simulink model "Commando2"  (R2012b)
settings: Solver=ode5  StartTime=0.0  StopTime=inf  FixedStep=sample_time  RelTol=1e-3
InitFcn:
  | sample_time=0.005;%0.004;%0.0025;%0.02;
  | sample_time_Vicon = 0.005;
  | DeltaT = 0.02;
  | g = 9.81;
  | H0 = g%0.3165;
  | Kl = 1;
  | 
  | Q6_mass = 0.8;
  | 
  | Q6_Omega_r = 1.2; %for horizon ref
  | Q6_Zeta_r = 0.707; %for horizon ref
  | Q6_Omega_r_h = 2;%for vertical ref
  | Q6_Zeta_r_h = 0.7; %for vertical ref
  | 
  | 
  | Q6_Omega = 1.3; %for horizon control
  | Q6_Zeta = 0.707; %for horizon control
  | Q6_Omega_h= 2; %for vertical control
  | Q6_Zeta_h = 0.7; %for vertical control
  | 
  | 
  | Q6_acc_max = 5;%horizontal max acc
  | Q6_acc_max_h = 5;%horizontal max acc
  | 
  | omega_circle = 30*pi/180;
  | 
  | omega_h = 0.1;%Ascending speed
  | PI = pi;
  | Circle_R = 1.9;
  | 
  | 
  | MAX_Height = -2;
  | 
  | 
  | % for NN
  | n = 5;
  | r = 3;
  | n2 = 5;
  | NN_ST = 0.02;
  | 
  | GAMA_V = 6;
  | gama_V_e = 0.01;
  | 
  | GAMA_W = GAMA_V;
  | gama_W_e =0.01;
  | 
  | % deadzone
  | NN_Deadzone_Z = 0;
  | 
  | % inputs nomalizaton parameters
  | NN_Z_y_min = -3;
  | NN_Z_y_max = 0.5;
  | 
  | NN_Z_v_max = 8;
  | NN_Z_v_min = -NN_Z_v_max;
  | 
  | % alpha = 0.034;
  | alpha = 1;
  | % c_f = 0.0015;
  | c_f = 0.001;
  | ... (+1 lines)
libraries: X330_Control x20, simulink x10
(part 2 of 2)

== stateflow chart Commando2/UAV 4/Trajectory Logic/UAV4 SF ==
  state Airborne
    state StopPoint2
      en:PosDesired = Pos;
    state TakeOff
      du:HoverThrottle = (H0 - HoverThrottle)*2*DeltaT + HoverThrottle ;
      PosDesired[2] = (-1.2 - PosDesired[2])*1*DeltaT + PosDesired[2] ;
    state StartPoint1
      en:PosDesired[0] = Circle_R*sin(270*PI/180 );
      PosDesired[1] = Circle_R*cos(270*PI/180);
    state StopPoint
      en:PosDesired = Pos;
      PosDesired[2]=-3;
    state StopPoint1
      en:
      PosDesired[0]=-2.2;
      PosDesired[1]=-2;
    state Circle2D
      du: PosDesired[0] = Circle_R*sin(270*PI/180 + T_circle*omega_circle);
      PosDesired[1] = Circle_R*cos(270*PI/180 + T_circle*omega_circle);
      PosDesired[2]=height;
      T_circle = T_circle + DeltaT;
    (default) -> TakeOff : {PosDesired = Pos; }
    Circle2D -> StopPoint2 [order 1] : [QD==1]
    StopPoint2 -> Circle2D : [QD==0]
    TakeOff -> StartPoint1 : after(10, sec)
    StartPoint1 -> Circle2D : [RC[5] > 0.5]
        | {T_circle = 0.0;}
    Circle2D -> StopPoint [order 2] : [RC[5] < 0.5]
    StopPoint -> StopPoint1 : after (3,sec)
  state Landing
    state Decsending
      en:PosDesired = Pos;
      du:PosDesired[2] = (0.2 - PosDesired[2])*1*DeltaT + PosDesired[2] ;
    state CutThrottle
      du:HoverThrottle = (0.0 - HoverThrottle)*5*DeltaT + HoverThrottle ;
    (default) -> Decsending
    Decsending -> CutThrottle : [Pos[2] > -0.2]
  Landing -> Airborne : [RC[6] > 0.5]
  Airborne -> Landing : [RC[6] < -0.5]
  (default) -> Landing : {HoverThrottle=0.0;}
  data: PosDesired output double size=4; HoverThrottle output double size=1; Mode output uint8 size=3; RC input size=8; Pos input size=4; height input size=1; DeltaT parameter size=1; H0 parameter size=1; Kl parameter size=1; VelCmd local double size=2 =0; line_count local int8 size=1 =0; triangle_count local int8 size=1 =0; T_circle local double size=1; omega_circle parameter size=1; PI parameter size=1; omega_h parameter size=1; Circle_R parameter size=1; MAX_Height parameter size=1; PosError output double; QD input double size=1

== stateflow chart Commando2/UAV 1/Trajectory Logic/UAV SF1 ==
  state Airborne
    state StopPoint2
      en:PosDesired = Pos;
    state TakeOff
      du:HoverThrottle = (H0 - HoverThrottle)*2*DeltaT + HoverThrottle ;
      PosDesired[2] = (-1.2 - PosDesired[2])*1*DeltaT + PosDesired[2] ;
    state StartPoint1
      en:PosDesired[0] = Circle_R*sin(0*PI/180 );
      PosDesired[1] = Circle_R*cos(0*PI/180);
    state StopPoint
      en:PosDesired = Pos;
      PosDesired[2]=-1.5;
    state Circle2D
      du: PosDesired[0] = Circle_R*sin(0*PI/180 + T_circle*omega_circle);
      PosDesired[1] = Circle_R*cos(0*PI/180 + T_circle*omega_circle);
      PosDesired[2]=height;
      T_circle = T_circle + DeltaT;
    state StopPoint1
      en:
      PosDesired[0]=-2.2;
      PosDesired[1]=1;
    (default) -> TakeOff : {PosDesired = Pos; }
    Circle2D -> StopPoint2 [order 1] : [QD==1]
    TakeOff -> StartPoint1 : after(5, sec)
    StopPoint2 -> Circle2D : [QD==0]
    StartPoint1 -> Circle2D : [RC[5] > 0.5]
        | {T_circle = 0.0;}
    Circle2D -> StopPoint [order 2] : [RC[5] < 0.5]
    StopPoint -> StopPoint1 : after (3, sec)
  state Landing
    state Decsending
      en:PosDesired = Pos;
      du:PosDesired[2] = (0.2 - PosDesired[2])*1*DeltaT + PosDesired[2] ;
    state CutThrottle
      du:HoverThrottle = (0.0 - HoverThrottle)*5*DeltaT + HoverThrottle ;
    (default) -> Decsending
    Decsending -> CutThrottle : [Pos[2] > -0.2]
  Landing -> Airborne : [RC[6] > 0.5]
  Airborne -> Landing : [RC[6] < -0.5]
  (default) -> Landing : {HoverThrottle=0.0;}
  data: PosDesired output double size=4; HoverThrottle output double size=1; Mode output uint8 size=3; RC input size=8; Pos input size=4; height input size=1; DeltaT parameter size=1; H0 parameter size=1; Kl parameter size=1; VelCmd local double size=2 =0; line_count local int8 size=1 =0; triangle_count local int8 size=1 =0; T_circle local double size=1; omega_circle parameter size=1; PI parameter size=1; omega_h parameter; Circle_R parameter size=1; MAX_Height parameter size=1; PosError output double; QD input double size=1
